simulink model "controlePorP"  (R2023a)
settings: Solver=VariableStepAuto  StartTime=0.0  StopTime=2800  RelTol=1e-3
values from neighbouring files (symbols this model uses):
  F2 = 6.32    [ConstantesCPQ23m.m]    (also in lugardasRaizes.m)
  K = J/(Tau*wn2)    [ConstantesCPQ23m.m]    (also in lugardasRaizes.m)
  qsi = (P/Tau)/(2*wn)    [ConstantesCPQ23m.m]    (also in lugardasRaizes.m)
  wn = sqrt(1/Tau)    [ConstantesCPQ23m.m]    (also in lugardasRaizes.m)
  wn2 = (1/Tau)    [ConstantesCPQ23m.m]    (also in lugardasRaizes.m)
settings Model: Creator=Estudo  LastModifiedBy=Estudo

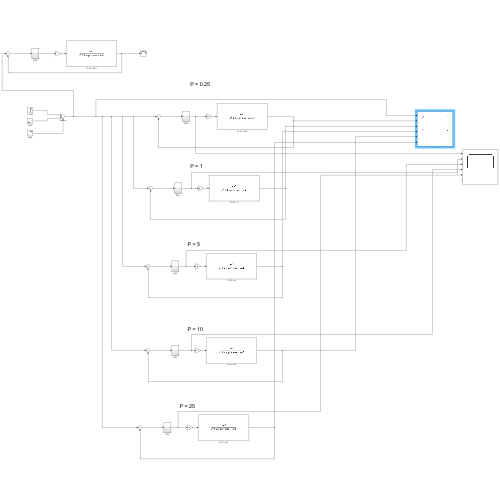
[thumbnail: Simulink's stored preview of the top-level diagram]
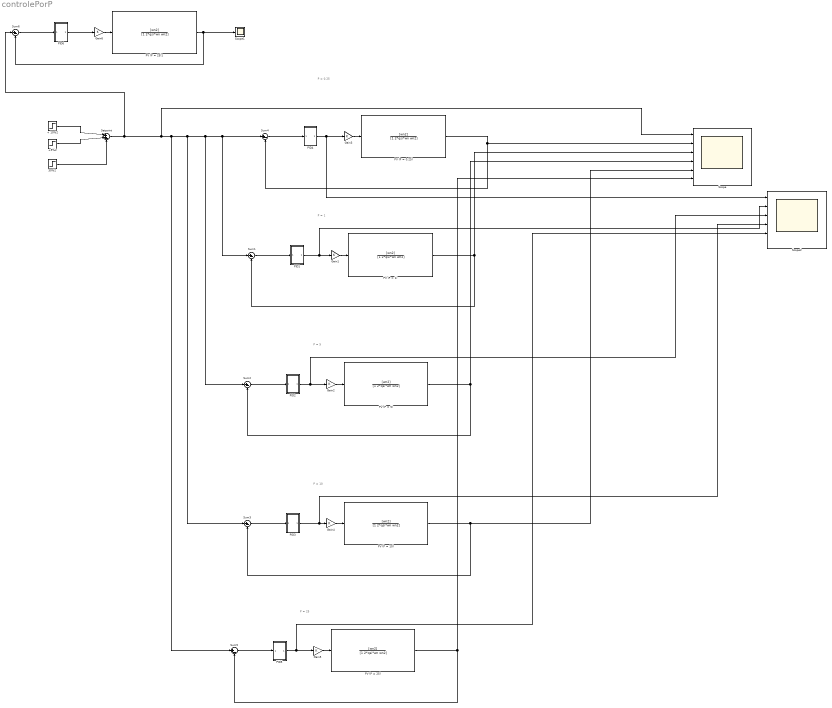
== system controlePorP ==
  note: P = 0.25
  note: P = 1
  note: P = 5
  note: P = 10
  note: P = 25
  + 10%2 : Step  After=F2 + F2*0.1  SampleTime=0
  +5%2 : Step  Time=1200  After=F2*0.05  SampleTime=0
  30%2 : Step  Time=2000  After=F2*0.3  SampleTime=0
  Gain{1..6} (6 alike) : Gain  Gain=K
  PID1 : Subsystem
  PID2 : Subsystem
  PID3 : Subsystem
  PID4 : Subsystem
  PID5 : Subsystem
  PID6 : Subsystem
  PV (P = 0.25) : TransferFcn  Numerator=[wn2]  Denominator=[1 2*qsi*wn wn2]
  PV (P = 1) : TransferFcn  Numerator=[wn2]  Denominator=[1 2*qsi*wn wn2]
  PV (P = 10) : TransferFcn  Numerator=[wn2]  Denominator=[1 2*qsi*wn wn2]
  PV (P = 25) : TransferFcn  Numerator=[wn2]  Denominator=[1 2*qsi*wn wn2]
  PV (P = 25)1 : TransferFcn  Numerator=[wn2]  Denominator=[1 2*qsi*wn wn2]
  PV (P = 5) : TransferFcn  Numerator=[wn2]  Denominator=[1 2*qsi*wn wn2]
  Scope : Scope  NumInputPorts=6
  Scope1 : Scope
  Scope2 : Scope  NumInputPorts=6
  Setpoint : Sum  Inputs=|++-
  Sum{1..6} (6 alike) : Sum  Inputs=|+-
  wires:
  +5%2/1 -> Setpoint/2
  30%2/1 -> Setpoint/3
  + 10%2/1 -> Setpoint/1
  PID4/1(Out1) -> Scope2/1, Gain3/1
  Gain3/1 -> PV (P = 0.25)/1
  Sum4/1 -> PID4/1(In1)
  PV (P = 0.25)/1 -> Scope/2, Sum4/2
  PID1/1(Out1) -> Scope2/2, Gain1/1
  Sum1/1 -> PID1/1(In1)
  PV (P = 1)/1 -> Scope/3, Sum1/2
  Gain1/1 -> PV (P = 1)/1
  Gain2/1 -> PV (P = 5)/1
  PV (P = 5)/1 -> Scope/4, Sum2/2
  Sum2/1 -> PID2/1(In1)
  PID2/1(Out1) -> Scope2/3, Gain2/1
  Gain4/1 -> PV (P = 10)/1
  PV (P = 10)/1 -> Scope/5, Sum3/2
  Sum3/1 -> PID3/1(In1)
  PID3/1(Out1) -> Scope2/4, Gain4/1
  Gain5/1 -> PV (P = 25)/1
  PV (P = 25)/1 -> Scope/6, Sum5/2
  Sum5/1 -> PID5/1(In1)
  Setpoint/1 -> Sum6/1, Scope/1, Sum5/1, Sum3/1, Sum2/1, Sum1/1, Sum4/1
  PID6/1(Out1) -> Gain6/1
  Sum6/1 -> PID6/1(In1)
  Gain6/1 -> PV (P = 25)1/1
  PV (P = 25)1/1 -> Scope1/1, Sum6/2
  PID5/1(Out1) -> Scope2/5, Gain5/1

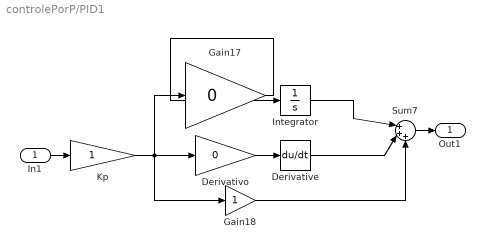
== system controlePorP/PID1 ==
  In1 : Inport
  Derivative : Derivative
  Derivativo : Gain  Gain=0
  Gain17 : Gain  Gain=0
  Gain18 : Gain
  Integrator : Integrator
  Kp : Gain
  Sum7 : Sum  Inputs=|+++
  Out1 : Outport
  wires:
  Gain18/1 -> Sum7/3
  Integrator/1 -> Sum7/1
  Kp/1 -> Gain17/1, Gain18/1, Derivativo/1
  Derivativo/1 -> Derivative/1
  In1/1 -> Kp/1
  Gain17/1 -> Integrator/1
  Derivative/1 -> Sum7/2
  Sum7/1 -> Out1/1

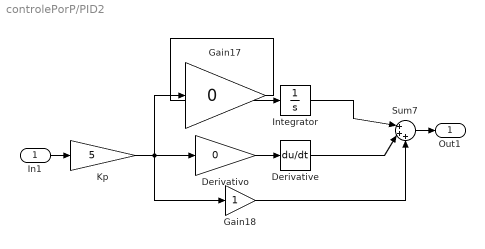
== system controlePorP/PID2 ==
  In1 : Inport
  Derivative : Derivative
  Derivativo : Gain  Gain=0
  Gain17 : Gain  Gain=0
  Gain18 : Gain
  Integrator : Integrator
  Kp : Gain  Gain=5
  Sum7 : Sum  Inputs=|+++
  Out1 : Outport
  wires:
  Gain18/1 -> Sum7/3
  Integrator/1 -> Sum7/1
  Kp/1 -> Gain17/1, Gain18/1, Derivativo/1
  Derivativo/1 -> Derivative/1
  In1/1 -> Kp/1
  Gain17/1 -> Integrator/1
  Derivative/1 -> Sum7/2
  Sum7/1 -> Out1/1

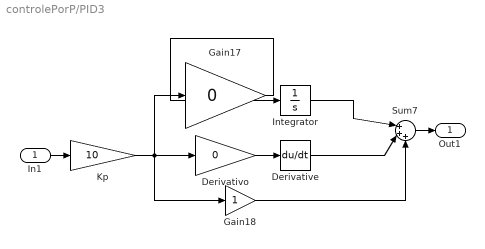
== system controlePorP/PID3 ==
  In1 : Inport
  Derivative : Derivative
  Derivativo : Gain  Gain=0
  Gain17 : Gain  Gain=0
  Gain18 : Gain
  Integrator : Integrator
  Kp : Gain  Gain=10
  Sum7 : Sum  Inputs=|+++
  Out1 : Outport
  wires:
  Gain18/1 -> Sum7/3
  Integrator/1 -> Sum7/1
  Kp/1 -> Gain17/1, Gain18/1, Derivativo/1
  Derivativo/1 -> Derivative/1
  In1/1 -> Kp/1
  Gain17/1 -> Integrator/1
  Derivative/1 -> Sum7/2
  Sum7/1 -> Out1/1

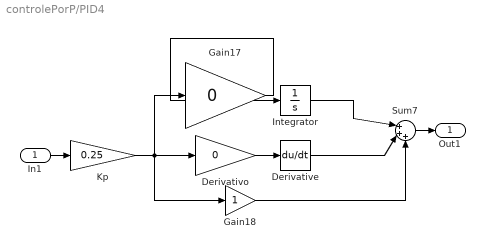
== system controlePorP/PID4 ==
  In1 : Inport
  Derivative : Derivative
  Derivativo : Gain  Gain=0
  Gain17 : Gain  Gain=0
  Gain18 : Gain
  Integrator : Integrator
  Kp : Gain  Gain=0.25
  Sum7 : Sum  Inputs=|+++
  Out1 : Outport
  wires:
  Gain18/1 -> Sum7/3
  Integrator/1 -> Sum7/1
  Kp/1 -> Gain17/1, Gain18/1, Derivativo/1
  Derivativo/1 -> Derivative/1
  In1/1 -> Kp/1
  Gain17/1 -> Integrator/1
  Derivative/1 -> Sum7/2
  Sum7/1 -> Out1/1

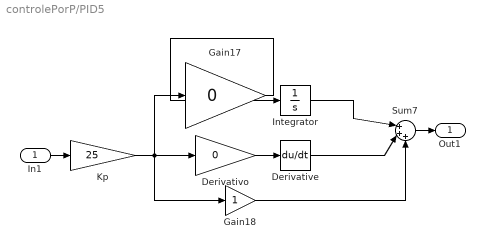
== system controlePorP/PID5 ==
  In1 : Inport
  Derivative : Derivative
  Derivativo : Gain  Gain=0
  Gain17 : Gain  Gain=0
  Gain18 : Gain
  Integrator : Integrator
  Kp : Gain  Gain=25
  Sum7 : Sum  Inputs=|+++
  Out1 : Outport
  wires:
  Gain18/1 -> Sum7/3
  Integrator/1 -> Sum7/1
  Kp/1 -> Gain17/1, Gain18/1, Derivativo/1
  Derivativo/1 -> Derivative/1
  In1/1 -> Kp/1
  Gain17/1 -> Integrator/1
  Derivative/1 -> Sum7/2
  Sum7/1 -> Out1/1

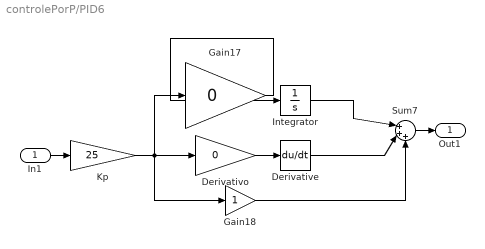
== system controlePorP/PID6 ==
  In1 : Inport
  Derivative : Derivative
  Derivativo : Gain  Gain=0
  Gain17 : Gain  Gain=0
  Gain18 : Gain
  Integrator : Integrator
  Kp : Gain  Gain=25
  Sum7 : Sum  Inputs=|+++
  Out1 : Outport
  wires:
  Gain18/1 -> Sum7/3
  Integrator/1 -> Sum7/1
  Kp/1 -> Gain17/1, Gain18/1, Derivativo/1
  Derivativo/1 -> Derivative/1
  In1/1 -> Kp/1
  Gain17/1 -> Integrator/1
  Derivative/1 -> Sum7/2
  Sum7/1 -> Out1/1
